simulink model "che322tutorial4"  (R2017a)
settings: Solver=ode4  StartTime=0.0  StopTime=10.0  FixedStep=0.01  RelTol=1e-3
settings Model: Creator=majeedhu  LastModifiedBy=donaghy1

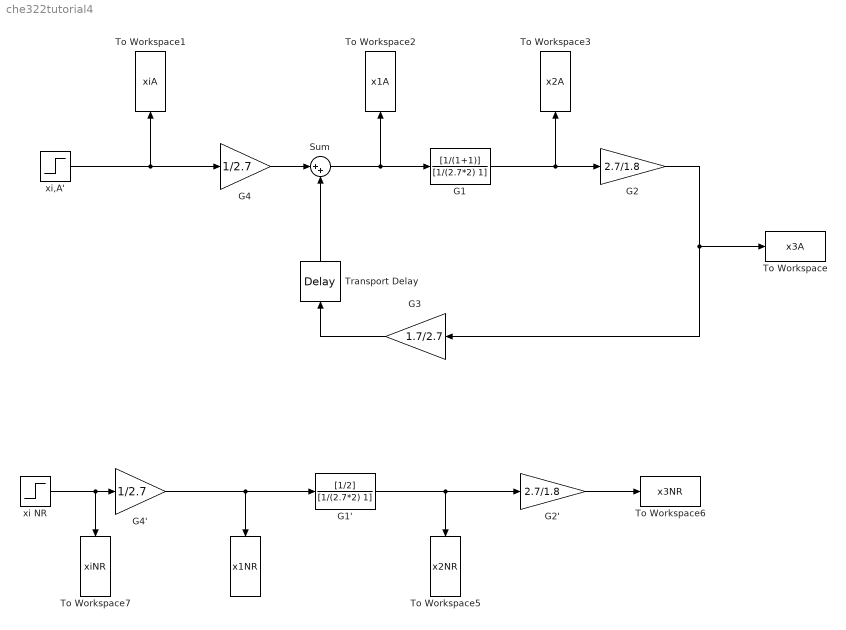
== system che322tutorial4 ==
  " " : ToWorkspace  VariableName=x1NR  SampleTime=-1
  G1 : TransferFcn  Numerator=[1/(1+1)]  Denominator=[1/(2.7*2) 1]
  G1' : TransferFcn  Numerator=[1/2]  Denominator=[1/(2.7*2) 1]
  G2 : Gain  Gain=2.7/1.8
  G2' : Gain  Gain=2.7/1.8
  "G3 " : Gain  Gain=1.7/2.7
  "G4 " : Gain  Gain=1/2.7
  G4' : Gain  Gain=1/2.7
  Sum : Sum  Inputs=|++
  To Workspace : ToWorkspace  VariableName=x3A  SampleTime=-1
  To Workspace1 : ToWorkspace  VariableName=xiA  SampleTime=-1
  To Workspace2 : ToWorkspace  VariableName=x1A  SampleTime=-1
  To Workspace3 : ToWorkspace  VariableName=x2A  SampleTime=-1
  To Workspace5 : ToWorkspace  VariableName=x2NR  SampleTime=-1
  To Workspace6 : ToWorkspace  VariableName=x3NR  SampleTime=-1
  To Workspace7 : ToWorkspace  VariableName=xiNR  SampleTime=-1
  Transport Delay : TransportDelay  DelayTime=0.1
  xi NR : Step  After=0.01  SampleTime=0
  xi,A' : Step  After=0.01  SampleTime=0
  wires:
  xi,A'/1 -> "G4 "/1, To Workspace1/1
  "G4 "/1 -> Sum/1
  G2/1 -> "G3 "/1, To Workspace/1
  Sum/1 -> To Workspace2/1, G1/1
  G1/1 -> G2/1, To Workspace3/1
  G4'/1 -> G1'/1, " "/1
  G1'/1 -> To Workspace5/1, G2'/1
  G2'/1 -> To Workspace6/1
  xi NR/1 -> G4'/1, To Workspace7/1
  "G3 "/1 -> Transport Delay/1
  Transport Delay/1 -> Sum/2
